simulink model "exp1_hover"  (R2020b)
settings: Solver=VariableStepAuto  StartTime=0.0  StopTime=30  FixedStep=0.01  RelTol=1e-3
values from neighbouring files (symbols this model uses):
  g = 9.8    [run_exp1.m]    (also in run_exp2.m; run_exp3_1.m; run_exp3_2.m)
  Ixx = 0.114    [run_exp1.m]    (also in run_exp2.m; run_exp3_1.m; run_exp3_2.m)
  Iyy = 0.114    [run_exp1.m]    (also in run_exp2.m; run_exp3_1.m; run_exp3_2.m)
  Izz = 0.158    [run_exp1.m]    (also in run_exp2.m; run_exp3_1.m; run_exp3_2.m)
  k_F = 6.11*10^(-8)*3600/(4*pi^2)    (= 5.57165188849e-06)    [run_exp1.m]    (also in run_exp2.m; run_exp3_1.m; run_exp3_2.m)
  k_M = 1.5*10^(-9)*3600/(4*pi^2)    (= 1.36783597917e-07)    [run_exp1.m]    (also in run_exp2.m; run_exp3_1.m; run_exp3_2.m)
  k_m = 20    [run_exp1.m]    (also in run_exp2.m; run_exp3_1.m; run_exp3_2.m)
  kd_phi = 4000    [run_exp1.m]    (also in run_exp2.m; run_exp3_1.m; run_exp3_2.m)
  kd_psi = 4000    [run_exp1.m]    (also in run_exp2.m; run_exp3_1.m; run_exp3_2.m)
  kd_theta = 4000    [run_exp1.m]    (also in run_exp2.m; run_exp3_1.m; run_exp3_2.m)
  kd_x = 1.0    (= 1)    [run_exp1.m]    (also in run_exp2.m; run_exp3_1.m; run_exp3_2.m)
  kd_y = 1.0    (= 1)    [run_exp1.m]    (also in run_exp2.m; run_exp3_1.m; run_exp3_2.m)
  kd_z = 2.0    (= 2)    [run_exp1.m]    (also in run_exp2.m; run_exp3_1.m; run_exp3_2.m)
  ki_x = 3e-4    (= 0.0003)    [run_exp1.m]    (also in run_exp2.m; run_exp3_1.m; run_exp3_2.m = 0.01)
  ki_y = 3e-4    (= 0.0003)    [run_exp1.m]    (also in run_exp2.m; run_exp3_1.m; run_exp3_2.m = 0.01)
  ki_z = 1e-6    (= 1e-06)    [run_exp1.m]    (also in run_exp2.m; run_exp3_1.m; run_exp3_2.m)
  kp_phi = 2000    [run_exp1.m]    (also in run_exp2.m; run_exp3_1.m; run_exp3_2.m)
  kp_psi = 800    [run_exp1.m]    (also in run_exp2.m; run_exp3_1.m; run_exp3_2.m)
  kp_theta = 2000    [run_exp1.m]    (also in run_exp2.m; run_exp3_1.m; run_exp3_2.m)
  kp_x = 0.5    [run_exp1.m]    (also in run_exp2.m; run_exp3_1.m; run_exp3_2.m = 1)
  kp_y = 0.5    [run_exp1.m]    (also in run_exp2.m; run_exp3_1.m; run_exp3_2.m = 1)
  kp_z = 1.2    [run_exp1.m]    (also in run_exp2.m; run_exp3_1.m; run_exp3_2.m)
  L = 0.2    [run_exp1.m]    (also in run_exp2.m; run_exp3_1.m; run_exp3_2.m)
  m = 0.5    [run_exp1.m]    (also in run_exp2.m; run_exp3_1.m; run_exp3_2.m)
  p_des = [10,10,-10]    [run_exp1.m]    (also in run_exp2.m)
libraries: pid_lib x6, shared6dof x1
settings Model: Creator=Yicheng Chen  LastModifiedBy=Yicheng Chen

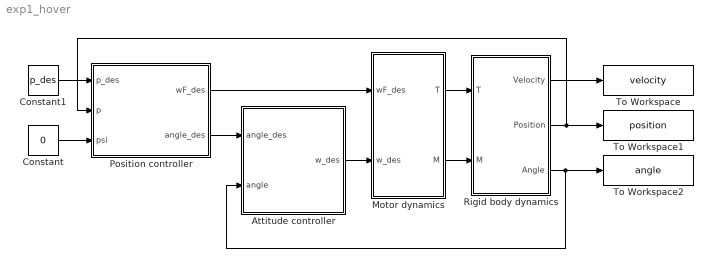
== system exp1_hover ==
  Attitude controller : Subsystem
  Constant : Constant  Value=0
  Constant1 : Constant  Value=p_des  VectorParams1D=off
  Motor dynamics : Subsystem
  Position controller : Subsystem
  Rigid body dynamics : Subsystem
  To Workspace : ToWorkspace  VariableName=velocity  SampleTime=-1
      settings: Save2DSignal=2-D array (concatenate along first dimension)
  To Workspace1 : ToWorkspace  VariableName=position  SampleTime=-1
      settings: Save2DSignal=2-D array (concatenate along first dimension)
  To Workspace2 : ToWorkspace  VariableName=angle  SampleTime=-1
      settings: Save2DSignal=2-D array (concatenate along first dimension)
  wires:
  Rigid body dynamics/1(Velocity) -> To Workspace/1
  Rigid body dynamics/2(Position) -> To Workspace1/1, Position controller/2(p)
  Rigid body dynamics/3(Angle) -> To Workspace2/1, Attitude controller/2(angle)
  Motor dynamics/1(T) -> Rigid body dynamics/1(T)
  Motor dynamics/2(M) -> Rigid body dynamics/2(M)
  Position controller/1(wF_des) -> Motor dynamics/1(wF_des)
  Position controller/2(angle_des) -> Attitude controller/1(angle_des)
  Constant1/1 -> Position controller/1(p_des)
  Constant/1 -> Position controller/3(psi)
  Attitude controller/1(w_des) -> Motor dynamics/2(w_des)

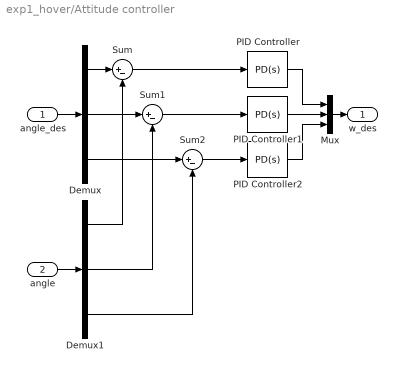
== system exp1_hover/Attitude controller ==
  angle_des : Inport
  angle : Inport  Port=2
  Demux : Demux  Outputs=3
  Demux1 : Demux  Outputs=3
  Mux : Mux  Inputs=3
  PID Controller : pid_lib/PID Controller  Controller=PD  Form=Parallel  TimeDomain=Continuous-time  UseExternalTs=off  SampleTime=-1  IntegratorMethod=Forward Euler  FilterMethod=Forward Euler  ControllerParametersSource=internal  P=kp_phi  I=1  D=kd_phi  UseFilter=on  N=100  TunerSelectOption=Transfer Function Based (PID Tuner App)  InitialConditionSource=internal  InitialConditionForIntegrator=0  InitialConditionForFilter=0  DifferentiatorICPrevScaledInput=0  ExternalReset=none  TrackingMode=off  Kt=1  LimitOutput=off  SatLimitsSource=internal  UpperSaturationLimit=inf  LowerSaturationLimit=-inf  LinearizeAsGain=on  AntiWindupMode=none  Kb=1  POutMin=[]  POutMax=[]  IOutMin=[]  IOutMax=[]  DOutMin=[]  DOutMax=[]  NOutMin=[]  NOutMax=[]  SumOutMin=[]  SumOutMax=[]  SaturationOutMin=[]  SaturationOutMax=[]  PParamMin=[]  PParamMax=[]  IParamMin=[]  IParamMax=[]  DParamMin=[]  DParamMax=[]  NParamMin=[]  NParamMax=[]  KbParamMin=[]  KbParamMax=[]  KtParamMin=[]  KtParamMax=[]  KbOutMin=[]  KbOutMax=[]  KtOutMin=[]  KtOutMax=[]  IntegratorOutMin=[]  IntegratorOutMax=[]  FilterOutMin=[]  FilterOutMax=[]  SumI1OutMin=[]  SumI1OutMax=[]  SumI2OutMin=[]  SumI2OutMax=[]  SumI3OutMin=[]  SumI3OutMax=[]  SumI4OutMin=[]  SumI4OutMax=[]  SumDOutMin=[]  SumDOutMax=[]  DifferentiatorOutMin=[]  DifferentiatorOutMax=[]  FilterDiffOutCoefMin=[]  FilterDiffOutCoefMax=[]  ReciprocalOutMin=[]  ReciprocalOutMax=[]  SumDenOutMin=[]  SumDenOutMax=[]  SumNumOutMin=[]  SumNumOutMax=[]  DivideOutMin=[]  DivideOutMax=[]  UdiffTsProdOutMin=[]  UdiffTsProdOutMax=[]  NTsProdOutMin=[]  NTsProdOutMax=[]  UintegralTsProdOutMin=[]  UintegralTsProdOutMax=[]  UngainTsProdOutMin=[]  UngainTsProdOutMax=[]  IntegratorContinuousStateAttributes=''  IntegratorStateMustResolveToSignalObject=off  IntegratorRTWStateStorageClass=Auto  FilterContinuousStateAttributes=''  FilterStateMustResolveToSignalObject=off  FilterRTWStateStorageClass=Auto  ParallelPVariant=InternalParameters  IdealPVariant=Disabled  IVariant=Disabled  DVariant=InternalParameters  IntegratorVariant=Disabled  SatVariant=Disabled  AWVariant=Disabled  PCopyVariant=Disabled  TRVariant=Disabled  FdbkBlocksVariant=Forward  IdealPFdbkVariant=Disabled  SatFdbkVariant=Disabled  DerivativeFilterVariant=ContFilter  NVariant=InternalParameters  NCopyVariant=Disabled  FilterICVariant=InternalICsFilter  IntegratorICVariant=Disabled  ExternalResetVariant=Disabled  TRSumVariant=Passthrough  SumFdbkVariant=Disabled  SumVariant=Sum_PD  TsampFilterVariant=InternalTs  TsampNgainVariant=Passthrough  TsampIntegralVariant=Disabled_SignalSpec  ExternalSaturationOutDataTypeStr=Inherit: Same as second input
  PID Controller1 : pid_lib/PID Controller  Controller=PD  Form=Parallel  TimeDomain=Continuous-time  UseExternalTs=off  SampleTime=-1  IntegratorMethod=Forward Euler  FilterMethod=Forward Euler  ControllerParametersSource=internal  P=kp_theta  I=1  D=kd_theta  UseFilter=on  N=100  TunerSelectOption=Transfer Function Based (PID Tuner App)  InitialConditionSource=internal  InitialConditionForIntegrator=0  InitialConditionForFilter=0  DifferentiatorICPrevScaledInput=0  ExternalReset=none  TrackingMode=off  Kt=1  LimitOutput=off  SatLimitsSource=internal  UpperSaturationLimit=inf  LowerSaturationLimit=-inf  LinearizeAsGain=on  AntiWindupMode=none  Kb=1  POutMin=[]  POutMax=[]  IOutMin=[]  IOutMax=[]  DOutMin=[]  DOutMax=[]  NOutMin=[]  NOutMax=[]  SumOutMin=[]  SumOutMax=[]  SaturationOutMin=[]  SaturationOutMax=[]  PParamMin=[]  PParamMax=[]  IParamMin=[]  IParamMax=[]  DParamMin=[]  DParamMax=[]  NParamMin=[]  NParamMax=[]  KbParamMin=[]  KbParamMax=[]  KtParamMin=[]  KtParamMax=[]  KbOutMin=[]  KbOutMax=[]  KtOutMin=[]  KtOutMax=[]  IntegratorOutMin=[]  IntegratorOutMax=[]  FilterOutMin=[]  FilterOutMax=[]  SumI1OutMin=[]  SumI1OutMax=[]  SumI2OutMin=[]  SumI2OutMax=[]  SumI3OutMin=[]  SumI3OutMax=[]  SumI4OutMin=[]  SumI4OutMax=[]  SumDOutMin=[]  SumDOutMax=[]  DifferentiatorOutMin=[]  DifferentiatorOutMax=[]  FilterDiffOutCoefMin=[]  FilterDiffOutCoefMax=[]  ReciprocalOutMin=[]  ReciprocalOutMax=[]  SumDenOutMin=[]  SumDenOutMax=[]  SumNumOutMin=[]  SumNumOutMax=[]  DivideOutMin=[]  DivideOutMax=[]  UdiffTsProdOutMin=[]  UdiffTsProdOutMax=[]  NTsProdOutMin=[]  NTsProdOutMax=[]  UintegralTsProdOutMin=[]  UintegralTsProdOutMax=[]  UngainTsProdOutMin=[]  UngainTsProdOutMax=[]  IntegratorContinuousStateAttributes=''  IntegratorStateMustResolveToSignalObject=off  IntegratorRTWStateStorageClass=Auto  FilterContinuousStateAttributes=''  FilterStateMustResolveToSignalObject=off  FilterRTWStateStorageClass=Auto  ParallelPVariant=InternalParameters  IdealPVariant=Disabled  IVariant=Disabled  DVariant=InternalParameters  IntegratorVariant=Disabled  SatVariant=Disabled  AWVariant=Disabled  PCopyVariant=Disabled  TRVariant=Disabled  FdbkBlocksVariant=Forward  IdealPFdbkVariant=Disabled  SatFdbkVariant=Disabled  DerivativeFilterVariant=ContFilter  NVariant=InternalParameters  NCopyVariant=Disabled  FilterICVariant=InternalICsFilter  IntegratorICVariant=Disabled  ExternalResetVariant=Disabled  TRSumVariant=Passthrough  SumFdbkVariant=Disabled  SumVariant=Sum_PD  TsampFilterVariant=InternalTs  TsampNgainVariant=Passthrough  TsampIntegralVariant=Disabled_SignalSpec  ExternalSaturationOutDataTypeStr=Inherit: Same as second input
  PID Controller2 : pid_lib/PID Controller  Controller=PD  Form=Parallel  TimeDomain=Continuous-time  UseExternalTs=off  SampleTime=-1  IntegratorMethod=Forward Euler  FilterMethod=Forward Euler  ControllerParametersSource=internal  P=kp_psi  I=1  D=kd_psi  UseFilter=on  N=100  TunerSelectOption=Transfer Function Based (PID Tuner App)  InitialConditionSource=internal  InitialConditionForIntegrator=0  InitialConditionForFilter=0  DifferentiatorICPrevScaledInput=0  ExternalReset=none  TrackingMode=off  Kt=1  LimitOutput=off  SatLimitsSource=internal  UpperSaturationLimit=inf  LowerSaturationLimit=-inf  LinearizeAsGain=on  AntiWindupMode=none  Kb=1  POutMin=[]  POutMax=[]  IOutMin=[]  IOutMax=[]  DOutMin=[]  DOutMax=[]  NOutMin=[]  NOutMax=[]  SumOutMin=[]  SumOutMax=[]  SaturationOutMin=[]  SaturationOutMax=[]  PParamMin=[]  PParamMax=[]  IParamMin=[]  IParamMax=[]  DParamMin=[]  DParamMax=[]  NParamMin=[]  NParamMax=[]  KbParamMin=[]  KbParamMax=[]  KtParamMin=[]  KtParamMax=[]  KbOutMin=[]  KbOutMax=[]  KtOutMin=[]  KtOutMax=[]  IntegratorOutMin=[]  IntegratorOutMax=[]  FilterOutMin=[]  FilterOutMax=[]  SumI1OutMin=[]  SumI1OutMax=[]  SumI2OutMin=[]  SumI2OutMax=[]  SumI3OutMin=[]  SumI3OutMax=[]  SumI4OutMin=[]  SumI4OutMax=[]  SumDOutMin=[]  SumDOutMax=[]  DifferentiatorOutMin=[]  DifferentiatorOutMax=[]  FilterDiffOutCoefMin=[]  FilterDiffOutCoefMax=[]  ReciprocalOutMin=[]  ReciprocalOutMax=[]  SumDenOutMin=[]  SumDenOutMax=[]  SumNumOutMin=[]  SumNumOutMax=[]  DivideOutMin=[]  DivideOutMax=[]  UdiffTsProdOutMin=[]  UdiffTsProdOutMax=[]  NTsProdOutMin=[]  NTsProdOutMax=[]  UintegralTsProdOutMin=[]  UintegralTsProdOutMax=[]  UngainTsProdOutMin=[]  UngainTsProdOutMax=[]  IntegratorContinuousStateAttributes=''  IntegratorStateMustResolveToSignalObject=off  IntegratorRTWStateStorageClass=Auto  FilterContinuousStateAttributes=''  FilterStateMustResolveToSignalObject=off  FilterRTWStateStorageClass=Auto  ParallelPVariant=InternalParameters  IdealPVariant=Disabled  IVariant=Disabled  DVariant=InternalParameters  IntegratorVariant=Disabled  SatVariant=Disabled  AWVariant=Disabled  PCopyVariant=Disabled  TRVariant=Disabled  FdbkBlocksVariant=Forward  IdealPFdbkVariant=Disabled  SatFdbkVariant=Disabled  DerivativeFilterVariant=ContFilter  NVariant=InternalParameters  NCopyVariant=Disabled  FilterICVariant=InternalICsFilter  IntegratorICVariant=Disabled  ExternalResetVariant=Disabled  TRSumVariant=Passthrough  SumFdbkVariant=Disabled  SumVariant=Sum_PD  TsampFilterVariant=InternalTs  TsampNgainVariant=Passthrough  TsampIntegralVariant=Disabled_SignalSpec  ExternalSaturationOutDataTypeStr=Inherit: Same as second input
  Sum : Sum  Inputs=|+-
  Sum1 : Sum  Inputs=|+-
  Sum2 : Sum  Inputs=|+-
  w_des : Outport
  wires:
  PID Controller/1 -> Mux/1
  PID Controller1/1 -> Mux/2
  Sum2/1 -> PID Controller2/1
  Sum/1 -> PID Controller/1
  PID Controller2/1 -> Mux/3
  Sum1/1 -> PID Controller1/1
  Demux/1 -> Sum/1
  Demux/2 -> Sum1/1
  Demux/3 -> Sum2/1
  angle_des/1 -> Demux/1
  angle/1 -> Demux1/1
  Demux1/1 -> Sum/2
  Demux1/2 -> Sum1/2
  Demux1/3 -> Sum2/2
  Mux/1 -> w_des/1

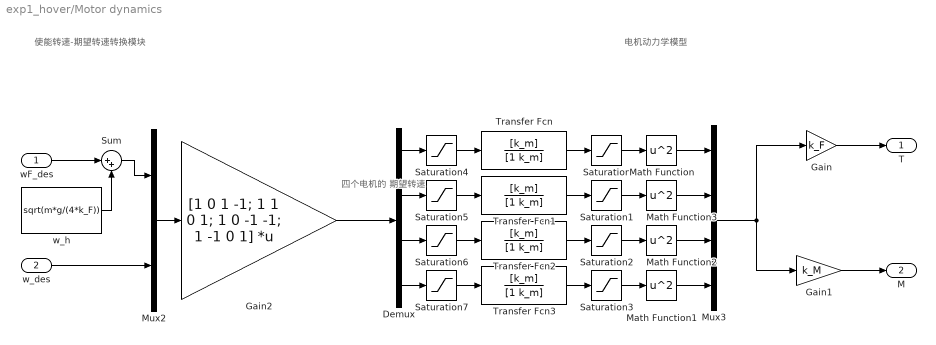
== system exp1_hover/Motor dynamics ==
  note: 四个电机的
      | 期望转速
  note: 电机动力学模型
  note: 使能转速-期望转速转换模块
  wF_des : Inport
  w_des : Inport  Port=2
  Demux : Demux
  Gain : Gain  Gain=k_F
  Gain1 : Gain  Gain=k_M
  Gain2 : Gain  Gain=[1 0 1 -1; 1 1 0 1; 1 0 -1 -1; 1 -1 0 1]  Multiplication=Matrix(K*u) (u vector)
  Math Function{,1..3} (4 alike) : Math  Operator=square  SaturateOnIntegerOverflow=on
  Mux2 : Mux  Inputs=2
  Mux3 : Mux
  Saturation{,1..7} (8 alike) : Saturate  UpperLimit=7800*2*pi/60  LowerLimit=1200*2*pi/60
  Sum : Sum  Inputs=|++
  Transfer Fcn{,1..3} (4 alike) : TransferFcn  Numerator=[k_m]  Denominator=[1 k_m]
  w_h : Constant  Value=sqrt(m*g/(4*k_F))
  T : Outport
  M : Outport  Port=2
  wires:
  Mux2/1 -> Gain2/1
  Sum/1 -> Mux2/1
  w_h/1 -> Sum/2
  Gain/1 -> T/1
  Mux3/1 -> Gain1/1, Gain/1
  Gain2/1 -> Demux/1
  Gain1/1 -> M/1
  wF_des/1 -> Sum/1
  Math Function/1 -> Mux3/1
  Math Function3/1 -> Mux3/2
  Math Function2/1 -> Mux3/3
  Math Function1/1 -> Mux3/4
  Transfer Fcn3/1 -> Saturation3/1
  Transfer Fcn/1 -> Saturation/1
  Transfer Fcn1/1 -> Saturation1/1
  Transfer Fcn2/1 -> Saturation2/1
  Saturation/1 -> Math Function/1
  Saturation3/1 -> Math Function1/1
  Saturation2/1 -> Math Function2/1
  Saturation1/1 -> Math Function3/1
  w_des/1 -> Mux2/2
  Saturation6/1 -> Transfer Fcn2/1
  Saturation7/1 -> Transfer Fcn3/1
  Saturation4/1 -> Transfer Fcn/1
  Saturation5/1 -> Transfer Fcn1/1
  Demux/1 -> Saturation4/1
  Demux/2 -> Saturation5/1
  Demux/3 -> Saturation6/1
  Demux/4 -> Saturation7/1

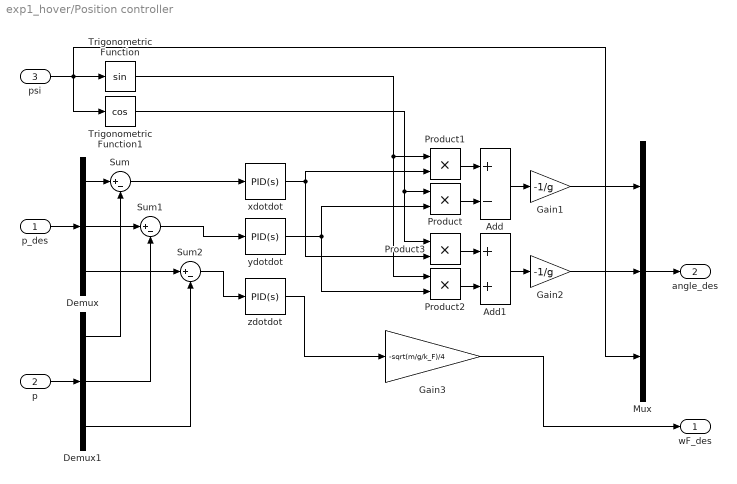
== system exp1_hover/Position controller ==
  p_des : Inport
  p : Inport  Port=2
  psi : Inport  Port=3
  Add : Sum  Inputs=+-
  Add1 : Sum
  Demux : Demux  Outputs=3
  Demux1 : Demux  Outputs=3
  Gain1 : Gain  Gain=-1/g
  Gain2 : Gain  Gain=-1/g
  Gain3 : Gain  Gain=-sqrt(m/g/k_F)/4
  Mux : Mux  Inputs=3
  Product{,1..3} (4 alike) : Product
  Sum : Sum  Inputs=|+-
  Sum1 : Sum  Inputs=|+-
  Sum2 : Sum  Inputs=|+-
  Trigonometric Function : Trigonometry
  Trigonometric Function1 : Trigonometry  Operator=cos
  xdotdot : pid_lib/PID Controller  Controller=PID  Form=Parallel  TimeDomain=Continuous-time  UseExternalTs=off  SampleTime=-1  IntegratorMethod=Forward Euler  FilterMethod=Forward Euler  ControllerParametersSource=internal  P=kp_x  I=ki_x  D=kd_x  UseFilter=on  N=100  TunerSelectOption=Transfer Function Based (PID Tuner App)  InitialConditionSource=internal  InitialConditionForIntegrator=0  InitialConditionForFilter=0  DifferentiatorICPrevScaledInput=0  ExternalReset=none  TrackingMode=off  Kt=1  LimitOutput=off  SatLimitsSource=internal  UpperSaturationLimit=inf  LowerSaturationLimit=-inf  LinearizeAsGain=on  AntiWindupMode=none  Kb=1  POutMin=[]  POutMax=[]  IOutMin=[]  IOutMax=[]  DOutMin=[]  DOutMax=[]  NOutMin=[]  NOutMax=[]  SumOutMin=[]  SumOutMax=[]  SaturationOutMin=[]  SaturationOutMax=[]  PParamMin=[]  PParamMax=[]  IParamMin=[]  IParamMax=[]  DParamMin=[]  DParamMax=[]  NParamMin=[]  NParamMax=[]  KbParamMin=[]  KbParamMax=[]  KtParamMin=[]  KtParamMax=[]  KbOutMin=[]  KbOutMax=[]  KtOutMin=[]  KtOutMax=[]  IntegratorOutMin=[]  IntegratorOutMax=[]  FilterOutMin=[]  FilterOutMax=[]  SumI1OutMin=[]  SumI1OutMax=[]  SumI2OutMin=[]  SumI2OutMax=[]  SumI3OutMin=[]  SumI3OutMax=[]  SumI4OutMin=[]  SumI4OutMax=[]  SumDOutMin=[]  SumDOutMax=[]  DifferentiatorOutMin=[]  DifferentiatorOutMax=[]  FilterDiffOutCoefMin=[]  FilterDiffOutCoefMax=[]  ReciprocalOutMin=[]  ReciprocalOutMax=[]  SumDenOutMin=[]  SumDenOutMax=[]  SumNumOutMin=[]  SumNumOutMax=[]  DivideOutMin=[]  DivideOutMax=[]  UdiffTsProdOutMin=[]  UdiffTsProdOutMax=[]  NTsProdOutMin=[]  NTsProdOutMax=[]  UintegralTsProdOutMin=[]  UintegralTsProdOutMax=[]  UngainTsProdOutMin=[]  UngainTsProdOutMax=[]  IntegratorContinuousStateAttributes=''  IntegratorStateMustResolveToSignalObject=off  IntegratorRTWStateStorageClass=Auto  FilterContinuousStateAttributes=''  FilterStateMustResolveToSignalObject=off  FilterRTWStateStorageClass=Auto  ParallelPVariant=InternalParameters  IdealPVariant=Disabled  IVariant=InternalParameters  DVariant=InternalParameters  IntegratorVariant=Continuous  SatVariant=Disabled  AWVariant=Passthrough  PCopyVariant=Disabled  TRVariant=Disabled  FdbkBlocksVariant=Forward  IdealPFdbkVariant=Disabled  SatFdbkVariant=Disabled  DerivativeFilterVariant=ContFilter  NVariant=InternalParameters  NCopyVariant=Disabled  FilterICVariant=InternalICsFilter  IntegratorICVariant=InternalICs  ExternalResetVariant=Disabled  TRSumVariant=Passthrough  SumFdbkVariant=Disabled  SumVariant=Sum_PID  TsampFilterVariant=InternalTs  TsampNgainVariant=Passthrough  TsampIntegralVariant=Passthrough  ExternalSaturationOutDataTypeStr=Inherit: Same as second input
  ydotdot : pid_lib/PID Controller  Controller=PID  Form=Parallel  TimeDomain=Continuous-time  UseExternalTs=off  SampleTime=-1  IntegratorMethod=Forward Euler  FilterMethod=Forward Euler  ControllerParametersSource=internal  P=kp_y  I=ki_y  D=kd_y  UseFilter=on  N=100  TunerSelectOption=Transfer Function Based (PID Tuner App)  InitialConditionSource=internal  InitialConditionForIntegrator=0  InitialConditionForFilter=0  DifferentiatorICPrevScaledInput=0  ExternalReset=none  TrackingMode=off  Kt=1  LimitOutput=off  SatLimitsSource=internal  UpperSaturationLimit=inf  LowerSaturationLimit=-inf  LinearizeAsGain=on  AntiWindupMode=none  Kb=1  POutMin=[]  POutMax=[]  IOutMin=[]  IOutMax=[]  DOutMin=[]  DOutMax=[]  NOutMin=[]  NOutMax=[]  SumOutMin=[]  SumOutMax=[]  SaturationOutMin=[]  SaturationOutMax=[]  PParamMin=[]  PParamMax=[]  IParamMin=[]  IParamMax=[]  DParamMin=[]  DParamMax=[]  NParamMin=[]  NParamMax=[]  KbParamMin=[]  KbParamMax=[]  KtParamMin=[]  KtParamMax=[]  KbOutMin=[]  KbOutMax=[]  KtOutMin=[]  KtOutMax=[]  IntegratorOutMin=[]  IntegratorOutMax=[]  FilterOutMin=[]  FilterOutMax=[]  SumI1OutMin=[]  SumI1OutMax=[]  SumI2OutMin=[]  SumI2OutMax=[]  SumI3OutMin=[]  SumI3OutMax=[]  SumI4OutMin=[]  SumI4OutMax=[]  SumDOutMin=[]  SumDOutMax=[]  DifferentiatorOutMin=[]  DifferentiatorOutMax=[]  FilterDiffOutCoefMin=[]  FilterDiffOutCoefMax=[]  ReciprocalOutMin=[]  ReciprocalOutMax=[]  SumDenOutMin=[]  SumDenOutMax=[]  SumNumOutMin=[]  SumNumOutMax=[]  DivideOutMin=[]  DivideOutMax=[]  UdiffTsProdOutMin=[]  UdiffTsProdOutMax=[]  NTsProdOutMin=[]  NTsProdOutMax=[]  UintegralTsProdOutMin=[]  UintegralTsProdOutMax=[]  UngainTsProdOutMin=[]  UngainTsProdOutMax=[]  IntegratorContinuousStateAttributes=''  IntegratorStateMustResolveToSignalObject=off  IntegratorRTWStateStorageClass=Auto  FilterContinuousStateAttributes=''  FilterStateMustResolveToSignalObject=off  FilterRTWStateStorageClass=Auto  ParallelPVariant=InternalParameters  IdealPVariant=Disabled  IVariant=InternalParameters  DVariant=InternalParameters  IntegratorVariant=Continuous  SatVariant=Disabled  AWVariant=Passthrough  PCopyVariant=Disabled  TRVariant=Disabled  FdbkBlocksVariant=Forward  IdealPFdbkVariant=Disabled  SatFdbkVariant=Disabled  DerivativeFilterVariant=ContFilter  NVariant=InternalParameters  NCopyVariant=Disabled  FilterICVariant=InternalICsFilter  IntegratorICVariant=InternalICs  ExternalResetVariant=Disabled  TRSumVariant=Passthrough  SumFdbkVariant=Disabled  SumVariant=Sum_PID  TsampFilterVariant=InternalTs  TsampNgainVariant=Passthrough  TsampIntegralVariant=Passthrough  ExternalSaturationOutDataTypeStr=Inherit: Same as second input
  zdotdot : pid_lib/PID Controller  Controller=PID  Form=Parallel  TimeDomain=Continuous-time  UseExternalTs=off  SampleTime=-1  IntegratorMethod=Forward Euler  FilterMethod=Forward Euler  ControllerParametersSource=internal  P=kp_z  I=ki_z  D=kd_z  UseFilter=on  N=100  TunerSelectOption=Transfer Function Based (PID Tuner App)  InitialConditionSource=internal  InitialConditionForIntegrator=0  InitialConditionForFilter=0  DifferentiatorICPrevScaledInput=0  ExternalReset=none  TrackingMode=off  Kt=1  LimitOutput=off  SatLimitsSource=internal  UpperSaturationLimit=inf  LowerSaturationLimit=-inf  LinearizeAsGain=on  AntiWindupMode=none  Kb=1  POutMin=[]  POutMax=[]  IOutMin=[]  IOutMax=[]  DOutMin=[]  DOutMax=[]  NOutMin=[]  NOutMax=[]  SumOutMin=[]  SumOutMax=[]  SaturationOutMin=[]  SaturationOutMax=[]  PParamMin=[]  PParamMax=[]  IParamMin=[]  IParamMax=[]  DParamMin=[]  DParamMax=[]  NParamMin=[]  NParamMax=[]  KbParamMin=[]  KbParamMax=[]  KtParamMin=[]  KtParamMax=[]  KbOutMin=[]  KbOutMax=[]  KtOutMin=[]  KtOutMax=[]  IntegratorOutMin=[]  IntegratorOutMax=[]  FilterOutMin=[]  FilterOutMax=[]  SumI1OutMin=[]  SumI1OutMax=[]  SumI2OutMin=[]  SumI2OutMax=[]  SumI3OutMin=[]  SumI3OutMax=[]  SumI4OutMin=[]  SumI4OutMax=[]  SumDOutMin=[]  SumDOutMax=[]  DifferentiatorOutMin=[]  DifferentiatorOutMax=[]  FilterDiffOutCoefMin=[]  FilterDiffOutCoefMax=[]  ReciprocalOutMin=[]  ReciprocalOutMax=[]  SumDenOutMin=[]  SumDenOutMax=[]  SumNumOutMin=[]  SumNumOutMax=[]  DivideOutMin=[]  DivideOutMax=[]  UdiffTsProdOutMin=[]  UdiffTsProdOutMax=[]  NTsProdOutMin=[]  NTsProdOutMax=[]  UintegralTsProdOutMin=[]  UintegralTsProdOutMax=[]  UngainTsProdOutMin=[]  UngainTsProdOutMax=[]  IntegratorContinuousStateAttributes=''  IntegratorStateMustResolveToSignalObject=off  IntegratorRTWStateStorageClass=Auto  FilterContinuousStateAttributes=''  FilterStateMustResolveToSignalObject=off  FilterRTWStateStorageClass=Auto  ParallelPVariant=InternalParameters  IdealPVariant=Disabled  IVariant=InternalParameters  DVariant=InternalParameters  IntegratorVariant=Continuous  SatVariant=Disabled  AWVariant=Passthrough  PCopyVariant=Disabled  TRVariant=Disabled  FdbkBlocksVariant=Forward  IdealPFdbkVariant=Disabled  SatFdbkVariant=Disabled  DerivativeFilterVariant=ContFilter  NVariant=InternalParameters  NCopyVariant=Disabled  FilterICVariant=InternalICsFilter  IntegratorICVariant=InternalICs  ExternalResetVariant=Disabled  TRSumVariant=Passthrough  SumFdbkVariant=Disabled  SumVariant=Sum_PID  TsampFilterVariant=InternalTs  TsampNgainVariant=Passthrough  TsampIntegralVariant=Passthrough  ExternalSaturationOutDataTypeStr=Inherit: Same as second input
  wF_des : Outport
  angle_des : Outport  Port=2
  wires:
  Demux/1 -> Sum/1
  Demux/2 -> Sum1/1
  Demux/3 -> Sum2/1
  Sum/1 -> xdotdot/1
  Demux1/2 -> Sum1/2
  Demux1/3 -> Sum2/2
  Demux1/1 -> Sum/2
  p_des/1 -> Demux/1
  p/1 -> Demux1/1
  Sum1/1 -> ydotdot/1
  Sum2/1 -> zdotdot/1
  psi/1 -> Trigonometric Function1/1, Mux/3, Trigonometric Function/1
  Mux/1 -> angle_des/1
  Gain1/1 -> Mux/1
  Add/1 -> Gain1/1
  Product1/1 -> Add/1
  Product/1 -> Add/2
  Product2/1 -> Add1/2
  Product3/1 -> Add1/1
  Add1/1 -> Gain2/1
  xdotdot/1 -> Product3/2, Product1/2
  Trigonometric Function/1 -> Product2/1, Product1/1
  ydotdot/1 -> Product2/2, Product/2
  Trigonometric Function1/1 -> Product3/1, Product/1
  Gain2/1 -> Mux/2
  zdotdot/1 -> Gain3/1
  Gain3/1 -> wF_des/1

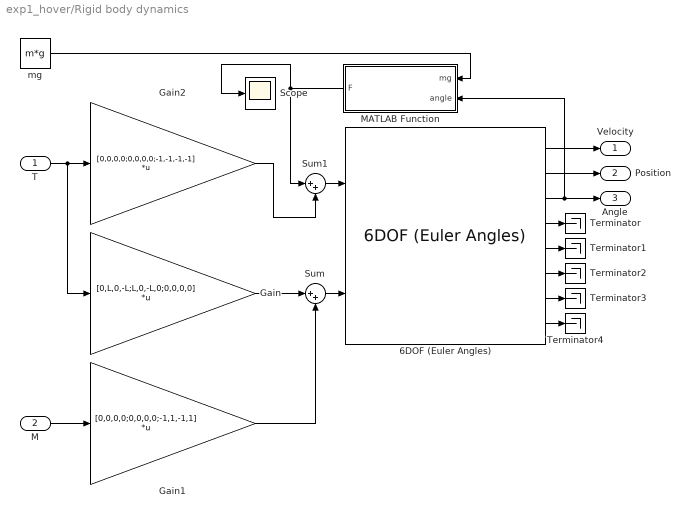
== system exp1_hover/Rigid body dynamics ==
  T : Inport
  M : Inport  Port=2
  6DOF (Euler Angles) : shared6dof/6DOF (Euler Angles)  units=Metric (MKS)  mtype=Fixed  rep=Euler Angles  xme_0=[0 0 0]  Vm_0=[0 0 0]  eul_0=[0 0 0]  pm_0=[0 0 0]  mass_0=m  mass_e=0.5  mass_f=2.0  inertia=[Ixx,0,0; 0,Iyy,0; 0,0,Izz]  inertia_e=eye(3)  inertia_f=2*eye(3)  k_quat=1.0  vre_flag=on  abi_flag=off  aMode=0  xme_statename=''  Vm_statename=''  eul_statename=''  quat_statename=''  pm_statename=''  mass_statename=''
      settings: SourceProductBaseCode=AE,PW,MT,UV,VE,VP
  Gain : Gain  Gain=[0,L,0,-L;L,0,-L,0;0,0,0,0]  Multiplication=Matrix(K*u) (u vector)
  Gain1 : Gain  Gain=[0,0,0,0;0,0,0,0;-1,1,-1,1]  Multiplication=Matrix(K*u) (u vector)
  Gain2 : Gain  Gain=[0,0,0,0;0,0,0,0;-1,-1,-1,-1]  Multiplication=Matrix(K*u) (u vector)
  MATLAB Function : MATLAB Function  TreatAsAtomicUnit=on
  Scope : Scope
  Sum : Sum  Inputs=|++
  Sum1 : Sum  Inputs=|++
  Terminator{,1..4} (5 alike) : Terminator
  mg : Constant  Value=m*g
  Velocity : Outport
  Position : Outport  Port=2
  Angle : Outport  Port=3
  wires:
  6DOF (Euler Angles)/1 -> Velocity/1
  T/1 -> Gain/1, Gain2/1
  6DOF (Euler Angles)/3 -> MATLAB Function/2(angle), Angle/1
  6DOF (Euler Angles)/2 -> Position/1
  Gain1/1 -> Sum/2
  Gain/1 -> Sum/1
  Sum/1 -> 6DOF (Euler Angles)/2
  M/1 -> Gain1/1
  Sum1/1 -> 6DOF (Euler Angles)/1
  Gain2/1 -> Sum1/2
  6DOF (Euler Angles)/4 -> Terminator/1
  6DOF (Euler Angles)/5 -> Terminator1/1
  6DOF (Euler Angles)/6 -> Terminator2/1
  6DOF (Euler Angles)/7 -> Terminator3/1
  6DOF (Euler Angles)/8 -> Terminator4/1
  mg/1 -> MATLAB Function/1(mg)
  MATLAB Function/1(F) -> Sum1/1, Scope/1

== matlab function exp1_hover/Rigid body dynamics/MATLAB Function ==
  data: mg input; angle input; F output
function F = mg_w2b(mg, angle)
phi = angle(1);
theta = angle(2);
F = [-sin(theta);cos(theta)*sin(phi);cos(phi)*cos(theta)] * mg;
